simulink model "EV_combined"  (R2024b)
settings: Solver=VariableStepAuto  StartTime=0.0  StopTime=100  RelTol=1e-3
libraries: spsDCVoltageSourceLib x2, spsDCMachineLib x1, sps_lib x1
settings Model: Creator=brain  LastModifiedBy=brain

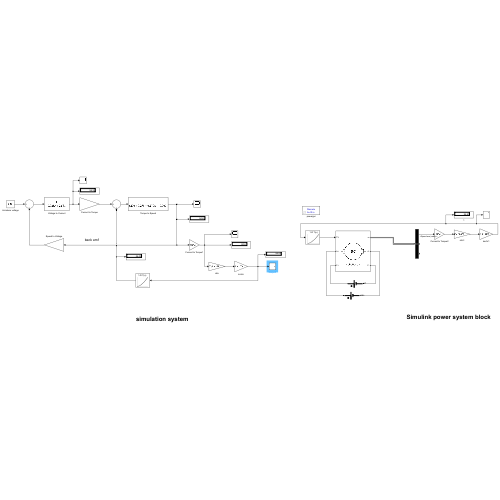
[thumbnail: Simulink's stored preview of the top-level diagram]
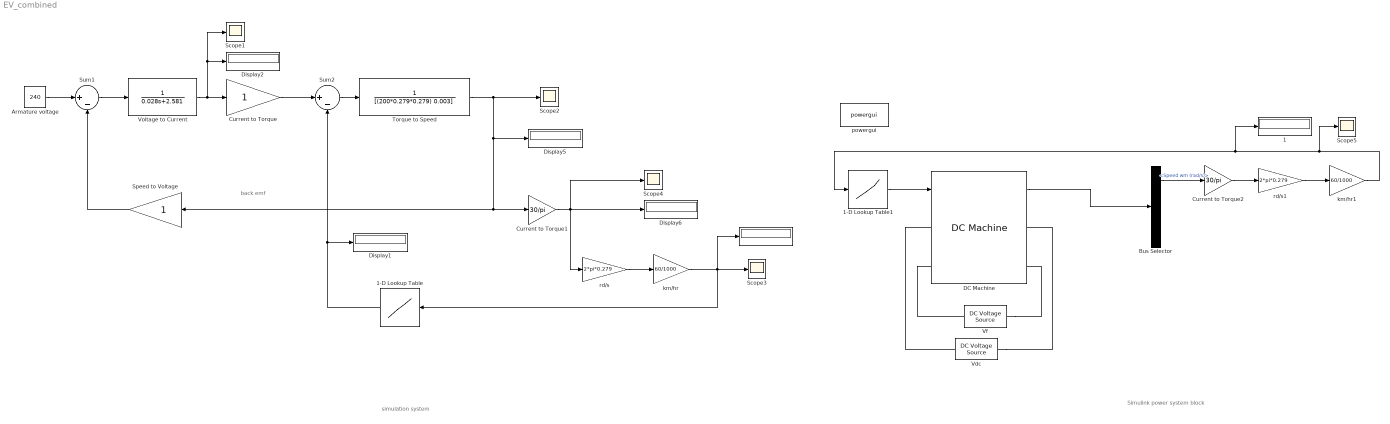
== system EV_combined ==
  note: Simulink power system block
  note: simulation system
  note: back emf
  " " : Display
  " 1" : Display
  1-D Lookup Table : Lookup_n-D  NumberOfTableDimensions=1  BreakpointsForDimension1=[28.4 56.8 63.5 69.56 75.13 80.32 85.19 89.8 94.19 98.37 102.4 106.3 110 113.6 117.1 120.5 123.8 127]  Table=[5 20 25 30 35 40 45 50 55 60 65 70 75 80 85 90 95 100]  InternalRulePriority=Speed  RndMeth=Simplest
  1-D Lookup Table1 : Lookup_n-D  NumberOfTableDimensions=1  BreakpointsForDimension1=[28.4 56.8 63.5 69.56 75.13 80.32 85.19 89.8 94.19 98.37 102.4 106.3 110 113.6 117.1 120.5 123.8 127]  Table=[5 20 25 30 35 40 45 50 55 60 65 70 75 80 85 90 95 100]  InternalRulePriority=Speed  RndMeth=Simplest
  Armature voltage : Constant  Value=240
  Bus Selector : BusSelector  OutputSignals=Speed wm (rad/s),Armature current ia (A),Electrical torque Te (n m)
  Current to Torque : Gain
  Current to Torque1 : Gain  Gain=30/pi
  Current to Torque2 : Gain  Gain=30/pi
  DC Machine : spsDCMachineLib/DC Machine  PresetModel=No  MechanicalLoad=Torque TL  FieldType=Wound  ShowDetailedParameters=on  MeasurementBus=off  RLa="[ 02.581  0.028]"  RLf="[ 281.3  3.156]"  Laf=0.9483  MachineConstant=Torque constant (N.m/A)  Ke=1.8  Kt=1.8  J=200*0.279*0.279  Bm=0.002953  Tf=0.5161  w0=1  Ifinit=1.06647707074298  TsPowergui=0  TsBlock=-1
  Display{1..2,5..6} (4 alike) : Display
  Scope{1..5} (5 alike) : Scope
  Speed to Voltage : Gain
  Sum1 : Sum  Inputs=|+-
  Sum2 : Sum  Inputs=|+-
  Torque to Speed : TransferFcn  Denominator=[(200*0.279*0.279) 0.003]
  Vdc : spsDCVoltageSourceLib/DC Voltage Source  Amplitude=240  Measurements=None
  Vf : spsDCVoltageSourceLib/DC Voltage Source  Amplitude=300  Measurements=None
  Voltage to Current : TransferFcn  Denominator=[0.028 2.581]
  km/hr : Gain  Gain=60/1000
  km/hr1 : Gain  Gain=60/1000
  powergui : sps_lib/powergui  Priority=1  SimulationMode=Discrete  SampleTime=50e-6  frequency=60  Iterations=50  frequencyindice=0  Pbase=100e6  ErrMax=1e-4  UnitsV=kV  UnitsW=MW  buscounter=0  FunctionMessages=off  echomessages=off  EnableUseOfTLC=off  CurrentSourceSwitches=off  DisableSnubberDevices=off  DisableRonSwitches=off  DisableVfSwitches=off  DisplayEquations=off  AutomaticDiscreteSolvers=off  SolverType=Tustin/Backward Euler (TBE)  Interpol=off  ExternalGateDelay=off  methode=off  Ts=100  x0status=blocks  SPID=on  SwTol=0  HookPort=off  NonlinearTolerance=1e-4  nMaxIteration=100  ContinueOnMaxIteration=off  RestoreLinks=warning  ResistiveCurrentMeasurement=off  Frange=[0:2:500]  Ylog=off  Xlog=on  ShowGrid=off  save=off  variable=ZData  structure=0  ZoomFFT=off  StartTime=0.0  cycles=1  DisplayStyle=1  fundamental=60  FreqAxis=off  MaxFrequency=1000  frequencyindicesteady=1  RmsSteady=1  display=off
  rd/s : Gain  Gain=2*pi*0.279
  rd/s1 : Gain  Gain=2*pi*0.279
  wires:
  Armature voltage/1 -> Sum1/1
  Voltage to Current/1 -> Display2/1, Scope1/1, Current to Torque/1
  Sum1/1 -> Voltage to Current/1
  Current to Torque1/1 -> Scope4/1, rd/s/1, Display6/1
  Sum2/1 -> Torque to Speed/1
  Speed to Voltage/1 -> Sum1/2
  Torque to Speed/1 -> Display5/1, Current to Torque1/1, Speed to Voltage/1, Scope2/1
  1-D Lookup Table/1 -> Display1/1, Sum2/2
  rd/s/1 -> km/hr/1
  km/hr/1 -> 1-D Lookup Table/1, Scope3/1, " "/1
  Current to Torque/1 -> Sum2/1
  1-D Lookup Table1/1 -> DC Machine/1
  DC Machine/1 -> Bus Selector/1
  Current to Torque2/1 -> rd/s1/1
  rd/s1/1 -> km/hr1/1
  km/hr1/1 -> Scope5/1, " 1"/1, 1-D Lookup Table1/1
  Bus Selector/1 -> Current to Torque2/1  "<Speed wm (rad/s)>"
  connections:
  Vf/RConn1 -- DC Machine/LConn2
  Vf/LConn1 -- DC Machine/RConn2
  Vdc/RConn1 -- DC Machine/LConn1
  Vdc/LConn1 -- DC Machine/RConn1
